simulink model "Encoder_Zynq_V25"  (R2021a)
settings: Solver=FixedStepDiscrete  StartTime=0.0  StopTime=SimulationsDauer  RelTol=1e-3
values from neighbouring files (symbols this model uses):
  f_ISR = 40e3    (= 40000)    [Script_Encoder_Zynq.m]
  IncPerTurn = 1024    [Script_Encoder_Zynq.m]
  inital_zero_speed_timeout = speed_timeout_in_s*f_fpga    (= 10000)    [Script_Encoder_Zynq.m]
  n_max = 6000    [Script_Encoder_Zynq.m]
  OmegaPerOverSampl = 500*((2*pi)/60)    (= 52.3598775598)    [Script_Encoder_Zynq.m]
  Periode = abs(1/Striche_pro_Sekunde)    [Script_Encoder_Zynq.m]
  Phase_Delay_A = Periode/8    [Script_Encoder_Zynq.m]
  Phase_Delay_B = -Periode/8    [Script_Encoder_Zynq.m]
  PolePair = 1    [Script_Encoder_Zynq.m]
  QuadratureFactor = 4    [Script_Encoder_Zynq.m]
  reciprocal_iterations = 3    [Script_Encoder_Zynq.m]
  T_50MHz = 1/f_50MHz    (= 1e-08)    [Script_Encoder_Zynq.m]
  T_mech = 1e-08    [Script_Encoder_Zynq.m]
undefined symbols (not defined in the file or in its folder): DiscIntNeverNeededParam, Newton, Raphson
libraries: hdlsllib x17, dspsrcs4 x3, simulink x2, dspswit3 x2, spsEdgeDetectorLib x2, simulink_extras x1, spspowerguiLib x1
(part 3 of 3)

== matlab function Encoder_Zynq_V25/IncreEncoder_V25/speed/oversampling factor logic/align_oversamples ==
  settings: fimath=fimath('RoundingMethod', 'Floor','OverflowAction', 'Wrap','ProductMode', 'FullPrecision', 'SumMode', 'FullPrecision')
  data: oversampling_factor input; A_state input; A_off output; Anot_state input; B_state input; Bnot_state input; Anot_off output; B_off output; Bnot_off output
function [A_off,Anot_off, B_off, Bnot_off] = fcn(oversampling_factor, A_state, Anot_state,B_state,Bnot_state)
    
%desired order A, B, notA, not B

% A_off    = fi(0, 0, 16, 0); 
% Anot_off = fi(0, 0, 16, 0); 
% B_off    = fi(0, 0, 16, 0); 
% Bnot_off = fi(0, 0, 16, 0); 

A_off    = logical(false); 
Anot_off = logical(false);
B_off    = logical(false);
Bnot_off = logical(false);


if (oversampling_factor>=2)
   %% A_state
    if(A_state == B_state)
        Anot_off =  logical(true);
    elseif(A_state == Anot_state)
        B_off =     logical(true);
    elseif(A_state == Bnot_state)
        Bnot_off =  logical(true);
    %% B_state
    elseif(B_state == Anot_state)
        B_off =     logical(true);
    elseif(B_state == Bnot_state)
        Bnot_off =  logical(true);
    %% Anot_state
    elseif(Anot_state == Bnot_state)
        Bnot_off =  logical(true);
    end
end


end

== matlab function Encoder_Zynq_V25/IncreEncoder_V25/speed/oversampling factor logic/Count ==
  settings: fimath=fimath('RoundingMethod', 'Floor','OverflowAction', 'Wrap','ProductMode', 'FullPrecision', 'SumMode', 'FullPrecision')
  data: AllowCheckOverSampl input; state_Out output fixdt(0,16,0); ReadBack_Omega input; OverSamplOmega input; state input fixdt(0,16,0); InternalOmega input; InternalOmega_Out output fixdt(1,24,11)
function [state_Out,InternalOmega_Out] = fcn(AllowCheckOverSampl, ReadBack_Omega,OverSamplOmega,state,InternalOmega)
    
 Fq16    = fimath('RoundingMethod', 'Floor', 'OverflowAction', 'Wrap','ProductMode', 'FullPrecision', 'ProductWordLength', 16,'ProductFractionLength',0,'SumMode','SpecifyPrecision','SumWordLength',16,'SumFractionLength',0);
%  Fq04    = fimath('RoundingMethod', 'Floor', 'OverflowAction', 'Wrap','ProductMode', 'FullPrecision', 'ProductWordLength', 4,'ProductFractionLength',0,'SumMode','SpecifyPrecision','SumWordLength',4,'SumFractionLength',0);
  Fq24    = fimath('RoundingMethod', 'Floor', 'OverflowAction', 'Wrap','ProductMode', 'FullPrecision', 'ProductWordLength', 24,'ProductFractionLength',11,'SumMode','SpecifyPrecision','SumWordLength',24,'SumFractionLength',11);


   %Counter for one measuring interval in order to trigger the ADC
    if isempty(InternalOmega)
        InternalOmega = fi(0, 1, 24, 11); 
    end

    %Counter State
    if isempty(state)
        state = fi(1, 0, 16, 0); 
    end
    
%% Count Up

     if (ReadBack_Omega > (InternalOmega + OverSamplOmega)) && (AllowCheckOverSampl == 1)
         state= fi(add(Fq16,state,fi(1, 0, 16, 0)),0,16,0);   %Count up the measure-state 
         InternalOmega = fi(add(Fq24,InternalOmega,OverSamplOmega),1,24,11);
     elseif(ReadBack_Omega < (InternalOmega - OverSamplOmega)) && (AllowCheckOverSampl == 1)
         state= fi(sub(Fq16,state,fi(1, 0, 16, 0)),0,16,0);   %Count up the measure-state 
         InternalOmega = fi(sub(Fq24,InternalOmega,OverSamplOmega),1,24,11);
     else
         state = state;
         InternalOmega= InternalOmega;
     end 

%% Output the variables 
    state_Out = state;
    InternalOmega_Out = InternalOmega;

end
